simulink model "simulation"  (R2024a)
settings: Solver=VariableStepAuto  StartTime=0.0  StopTime=0.10  RelTol=1e-3
libraries: spsDistributedParametersLineLib x2, spsRMSLib x2, spsThreePhaseSeriesRLCLoadLib x1, spsThreePhaseTransformerTwoWindingsLib x1, spsThreePhaseVIMeasurementLib x1, spsThreePhaseFaultLib x1, spsThreePhaseSourceLib x1, sps_lib x1
settings Model: Creator=Subash  LastModifiedBy=subed
settings DataIOCC: ReturnWorkspaceOutputs=off
settings OptimizationCC: ReuseModelBlockBuffer=off
settings RTWCC: GPUComputeCapability=3.5

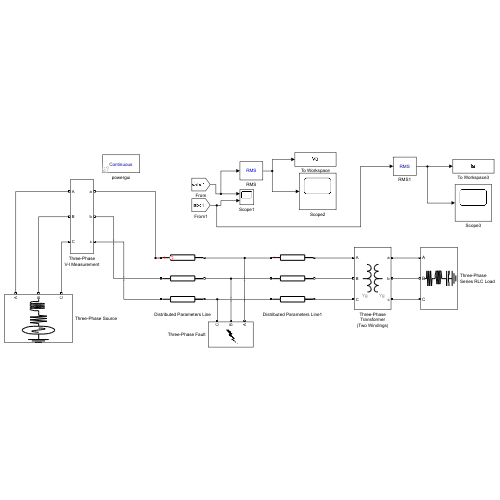
[thumbnail: Simulink's stored preview of the top-level diagram]
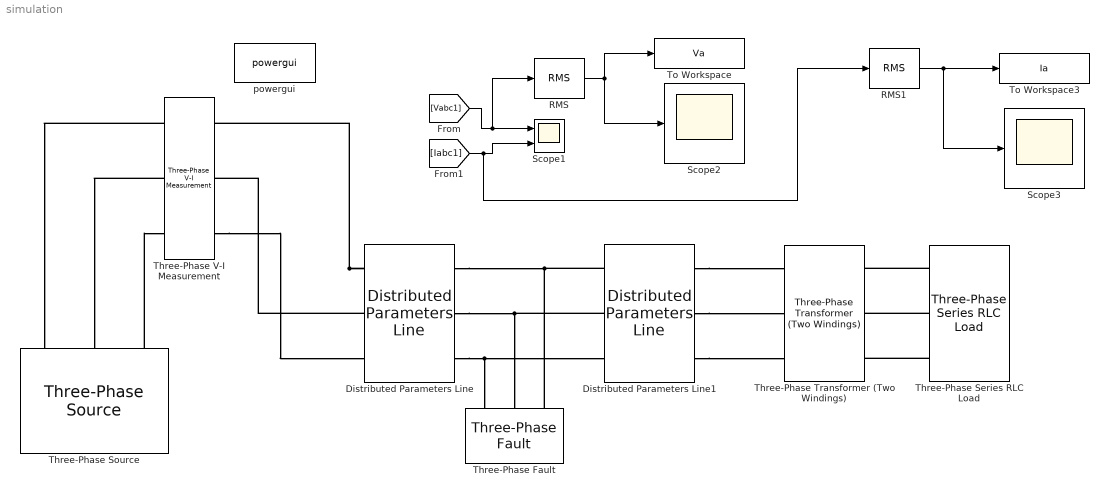
== system simulation ==
  Distributed Parameters Line : spsDistributedParametersLineLib/Distributed Parameters Line  Phases=3  Length=60  Frequency=50  Resistance=[0.01273 0.3864]  Inductance="[0.9337e-3  4.1264e-3]"  Capacitance=[12.74e-9 7.751e-9]  x1=[1.7470822706217e-11 24925.2353883314 24925.2353883314;314.159265358979 314.159265358979 314.159265358979;0.568138868293144 0.452394912356469 -1.11840141443843]  x2=[2.24158618637637e-10 24698.0495341447 24698.0495341446;314.159265358979 314.159265358979 314.159265358979;0.29349486364494 0.430509132540393 -1.1402871942545]  x3=[2.44946341274299e-12 61.3203954608641 61.3203954608682;314.159265358979 314.159265358979 314.159265358979;-0.989057405197225 0.597924748327279 -0.972871578467584]  x4=[2.49412211028762e-12 123.310110005917 123.310110005913;314.159265358979 314.159265358979 314.159265358979;1.97708012370418 0.315432433491663 -1.25536389330326]  x5=0.000339324940197446  V1=[1.747e-11 2.493e+04 2.493e+04;314.2 314.2 314.2;0.5681 0.4524 -1.118]  V2=[2.242e-10 2.47e+04 2.47e+04;314.2 314.2 314.2;0.2935 0.4305 -1.14]  I1=[2.449e-12 61.32 61.32;314.2 314.2 314.2;-0.9891 0.5979 -0.9729]  I2=[2.494e-12 123.3 123.3;314.2 314.2 314.2;1.977 0.3154 -1.255]  nHarmo=1  Measurements=None  Decoupling=off  VsMag0=0  VrMag0=0  VsAngle0=0  VrAngle0=0  IsMag0=0  IrMag0=0  IsAngle0=0  IrAngle0=0
      settings: LibrarySourceBlock=sps_lib/Power Grid Elements/Distributed Parameters Line
  Distributed Parameters Line1 : spsDistributedParametersLineLib/Distributed Parameters Line  Phases=3  Length=65  Frequency=50  Resistance=[0.01273 0.3864]  Inductance="[0.9337e-3  4.1264e-3]"  Capacitance=[12.74e-9 7.751e-9]  x1=[2.24158618637637e-10 24698.0495341447 24698.0495341446;314.159265358979 314.159265358979 314.159265358979;0.284611357484072 0.42509151589935 -1.14570481089554]  x2=[4.1919418863926e-10 24347.8248166446 24347.8248166445;314.159265358979 314.159265358979 314.159265358979;0.179504034269241 0.401225244676426 -1.16957108211846]  x3=[2.22392037119455e-12 61.4691074905795 61.469107490583;314.159265358979 314.159265358979 314.159265358979;-1.05471490486406 0.657491219597556 -0.913305107197309]  x4=[2.16414846619562e-12 122.944454954188 122.944454954185;314.159265358979 314.159265358979 314.159265358979;1.65017466639249 0.239635800626513 -1.3311605261684]  x5=0.000367602018547233  V1=[2.242e-10 2.47e+04 2.47e+04;314.2 314.2 314.2;0.2846 0.4251 -1.146]  V2=[4.192e-10 2.435e+04 2.435e+04;314.2 314.2 314.2;0.1795 0.4012 -1.17]  I1=[2.224e-12 61.47 61.47;314.2 314.2 314.2;-1.055 0.6575 -0.9133]  I2=[2.164e-12 122.9 122.9;314.2 314.2 314.2;1.65 0.2396 -1.331]  nHarmo=1  Measurements=None  Decoupling=off  VsMag0=0  VrMag0=0  VsAngle0=0  VrAngle0=0  IsMag0=0  IrMag0=0  IsAngle0=0  IrAngle0=0
      settings: LibrarySourceBlock=sps_lib/Power Grid Elements/Distributed Parameters Line
  RMS : spsRMSLib/RMS  TrueRMS=on  Freq=50  RMSInit=120  Ts=0
  RMS1 : spsRMSLib/RMS  TrueRMS=on  Freq=50  RMSInit=120  Ts=0
  Scope1 : Scope  NumInputPorts=2
  Scope2 : Scope
  Scope3 : Scope
  Three-Phase Series RLC Load : spsThreePhaseSeriesRLCLoadLib/Three-Phase Series RLC Load  LConnTagsString=A|B|C  Configuration=Y (grounded)  NominalVoltage=1000  Vabc=[1e3 1e3 1e3]  Vabcp=[1e3 1e3 1e3]  NominalFrequency=50  UnbalancedPower=off  ActivePower=10e3  InductivePower=100  CapacitivePower=100  Pabc=[10e3 9e3 11e3]  QLabc=[100 90 110]  QCabc=[100 90 110]  Pabcp=[10e3 9e3 11e3]  QLabcp=[100 90 110]  QCabcp=[100 90 110]  Measurements=None  LoadType=constant Z
  Three-Phase Transformer (Two Windings) : spsThreePhaseTransformerTwoWindingsLib/Three-Phase Transformer (Two Windings)  Winding1Connection=Yg  Winding2Connection=Yg  CoreType=Three single-phase transformers  SetSaturation=off  Hysteresis=off  DataFile='hysteresis'  SetInitialFlux=off  Measurements=None  UNITS=pu  NominalPower=[ 250e6 , 50 ]  Winding1=[ 735e3 , 0.002 , 0.08 ]  Winding2=[ 315e3 , 0.002 , 0.08 ]  Rm=500  Lm=500  L0=0.5  Saturation=[ 0,0 ; 0.0024,1.2 ; 1.0,1.52 ]  InitialFluxes=[ 0.8 , -0.8 , 0.7 ]  BreakLoop=off  DiscreteSolver=Trapezoidal iterative  DataType=off  TransfoNumber=1
  Three-Phase V-I Measurement : spsThreePhaseVIMeasurementLib/Three-Phase V-I Measurement  VoltageMeasurement=phase-to-phase  SetLabelV=on  LabelV=Vabc1  Vpu=off  VpuLL=off  CurrentMeasurement=yes  SetLabelI=on  LabelI=Iabc1  Ipu=off  Pbase=100e6  Vbase=500e3  OutputType=Complex  PhasorSimulation=off  PSBequivalent=0
  Three-Phase Fault : spsThreePhaseFaultLib/Three-Phase Fault  InitialStates=0  FaultA=on  FaultB=on  FaultC=off  GroundFault=on  SwitchTimes="[0.02  0.08]"  External=off  SwitchStatus=NaN  FaultResistance=0  GroundResistance=0.01  SnubberResistance=1e5  SnubberCapacitance=inf  Measurements=Fault voltages and currents
  Three-Phase Source : spsThreePhaseSourceLib/Three-Phase Source  InternalConnection=Yg  VoltagePhases=off  Voltage=25e3  PhaseAngle=0  Voltage_phases=[25e3 25e3 25e3]/sqrt(3)  PhaseAngles_phases=[0 -120 +120]  Frequency=50  NonIdealSource=on  SpecifyImpedance=off  Resistance=0.8929  Inductance=16.58e-3  ShortCircuitLevel=100e6  BaseVoltage=25e3  XRratio=7  BusType=swing  Pref=10e3  Qref=0  Prefabc=[10e3, 10e3, 10e3]  Qrefabc=[0, 0, 0]  Qmin=-inf  Qmax=inf
  To Workspace : ToWorkspace  VariableName=Va  SaveFormat=Structure With Time  SampleTime=-1
  To Workspace3 : ToWorkspace  VariableName=Ia  SaveFormat=Structure With Time  SampleTime=-1
  powergui : sps_lib/powergui  Priority=1  SimulationMode=Continuous  SampleTime=50e-6  frequency=60  Iterations=50  frequencyindice=50  Pbase=100e6  ErrMax=1e-4  UnitsV=kV  UnitsW=MW  buscounter=0  FunctionMessages=off  echomessages=off  EnableUseOfTLC=off  CurrentSourceSwitches=off  DisableSnubberDevices=off  DisableRonSwitches=off  DisableVfSwitches=off  DisplayEquations=off  AutomaticDiscreteSolvers=off  SolverType=Tustin/Backward Euler (TBE)  Interpol=off  ExternalGateDelay=off  methode=off  Ts=100  x0status=blocks  SPID=on  SwTol=0  HookPort=off  NonlinearTolerance=1e-4  nMaxIteration=100  ContinueOnMaxIteration=off  RestoreLinks=warning  ResistiveCurrentMeasurement=off  Frange=[0:2:500]  Ylog=off  Xlog=on  ShowGrid=off  save=off  variable=ZData  structure=0  ZoomFFT=off  StartTime=0.0  cycles=1  DisplayStyle=1  fundamental=60  FreqAxis=off  MaxFrequency=1000  frequencyindicesteady=1  RmsSteady=1  display=off
  wires:
  [Vabc1] -> RMS/1, Scope1/1
  [Iabc1] -> RMS1/1, Scope1/2
  RMS/1 -> To Workspace/1, Scope2/1
  RMS1/1 -> Scope3/1, To Workspace3/1
  connections:
  Distributed Parameters Line/RConn1 -- Distributed Parameters Line1/LConn1 -- Three-Phase Fault/LConn1
  Distributed Parameters Line/RConn2 -- Distributed Parameters Line1/LConn2 -- Three-Phase Fault/LConn2
  Distributed Parameters Line/RConn3 -- Distributed Parameters Line1/LConn3 -- Three-Phase Fault/LConn3
  Three-Phase Series RLC Load/LConn2 -- Three-Phase Transformer (Two Windings)/RConn2
  Three-Phase Series RLC Load/LConn3 -- Three-Phase Transformer (Two Windings)/RConn3
  Three-Phase Series RLC Load/LConn1 -- Three-Phase Transformer (Two Windings)/RConn1
  Distributed Parameters Line1/RConn1 -- Three-Phase Transformer (Two Windings)/LConn1
  Distributed Parameters Line1/RConn2 -- Three-Phase Transformer (Two Windings)/LConn2
  Distributed Parameters Line1/RConn3 -- Three-Phase Transformer (Two Windings)/LConn3
  Three-Phase V-I Measurement/LConn1 -- Three-Phase Source/RConn1
  Three-Phase V-I Measurement/LConn2 -- Three-Phase Source/RConn2
  Three-Phase Source/RConn3 -- Three-Phase V-I Measurement/LConn3
  Distributed Parameters Line/LConn1 -- Three-Phase V-I Measurement/RConn1
  Distributed Parameters Line/LConn2 -- Three-Phase V-I Measurement/RConn2
  Three-Phase V-I Measurement/RConn3 -- Distributed Parameters Line/LConn3
